simulink model "TPR_Ursino"  (Simulink 7.0)
settings: Solver=ode45  StartTime=0.0  StopTime=10.0  RelTol=1e-3
undefined symbols (not defined in the file or in its folder): Dx, ftas_min, Gas_sleep, initx, toux
settings Model: Creator=CLM  LastModifiedBy=CLM
settings OptimizationCC: BlockReduction=off  BooleanDataType=off
settings DebuggingCC: SaveWithParameterizedLinksMsg=none  SignalResolutionControl=TryResolveAllWithWarning  SolverPrmCheckMsg=none  MultiTaskDSMMsg=warning  MultiTaskCondExecSysMsg=none  StrictBusMsg=None
settings HardwareCC: TargetUnknown=on
settings RTWCC: IncludeERTFirstTime=on
settings GRTTargetCC: TargetFcnLib=ansi_tfl_tmw.mat

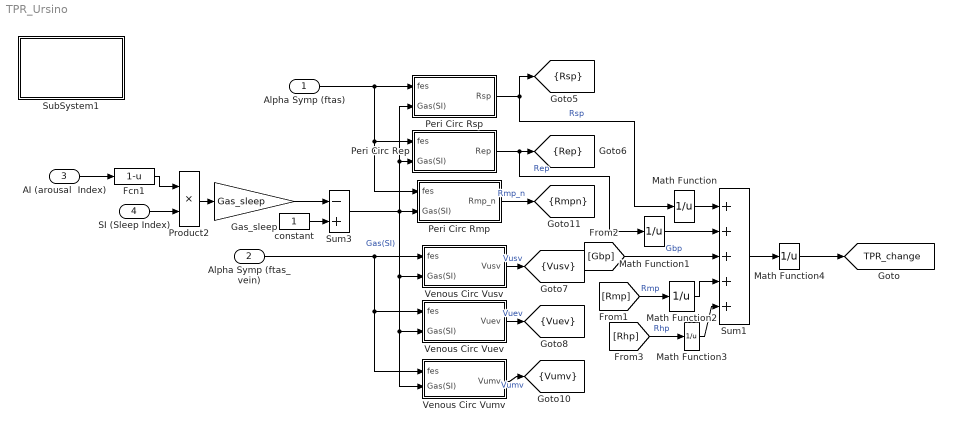
== system TPR_Ursino ==
  Alpha Symp (ftas) : Inport  OutDataType=sfix(16)  OutScaling=2^0
  Alpha Symp (ftas_vein) : Inport  Port=2  OutDataType=sfix(16)  OutScaling=2^0
  AI (arousal  Index) : Inport  Port=3  OutDataType=sfix(16)  OutScaling=2^0
  "SI (Sleep Index) " : Inport  Port=4  OutDataType=sfix(16)  OutScaling=2^0
  Fcn1 : Fcn  Expr=1-u
  Gas_sleep : Gain  Gain=Gas_sleep  ParameterDataType=sfix(16)  ParameterScaling=2^0  OutDataType=sfix(16)  OutScaling=2^0  SaturateOnIntegerOverflow=on
  Math Function{,1..4} (5 alike) : Math  Operator=reciprocal  OutDataType=sfix(16)  OutScaling=2^0  SaturateOnIntegerOverflow=on
  Peri Circ Rep : Subsystem
  Peri Circ Rmp : Subsystem
  Peri Circ Rsp : Subsystem
  Product2 : Product  OutDataType=sfix(16)  OutScaling=2^0  SaturateOnIntegerOverflow=on  InputSameDT=on
  SubSystem1 : Subsystem
      settings: OpenFcn=pneuma_variables
      mask Display: disp('"double click here"\n to load \nTPR_Ursino \ninitial values');
  Sum1 : Sum  Inputs=+++++  OutDataType=sfix(16)  OutScaling=2^0  SaturateOnIntegerOverflow=on  InputSameDT=on
  Sum3 : Sum  Inputs=-+  OutDataType=sfix(16)  OutScaling=2^0  SaturateOnIntegerOverflow=on  InputSameDT=on
  Venous Circ Vuev : Subsystem
  Venous Circ Vumv : Subsystem
  Venous Circ Vusv : Subsystem
  constant : Constant  OutDataType=sfix(16)  OutScaling=2^0
  tag scope: Rep=scoped, Rmpn=scoped, Rsp=scoped, TPR_change=global, Vuev=scoped, Vumv=scoped, Vusv=scoped
  wires:
  AI (arousal  Index)/1 -> Fcn1/1
  "SI (Sleep Index) "/1 -> Product2/2
  Fcn1/1 -> Product2/1
  Product2/1 -> Gas_sleep/1
  constant/1 -> Sum3/2
  Gas_sleep/1 -> Sum3/1
  Peri Circ Rep/1(Rep) -> [Rep], Math Function1/1  "Rep"
  Venous Circ Vusv/1(Vusv) -> [Vusv]  "Vusv"
  Venous Circ Vuev/1(Vuev) -> [Vuev]  "Vuev"
  Peri Circ Rsp/1(Rsp) -> [Rsp], Math Function/1  "Rsp"
  Venous Circ Vumv/1(Vumv) -> [Vumv]  "Vumv"
  Peri Circ Rmp/1(Rmp_n) -> [Rmpn]  "Rmp_n"
  Alpha Symp (ftas)/1 -> Peri Circ Rep/1(fes), Peri Circ Rmp/1(fes), Peri Circ Rsp/1(fes)
  Sum3/1 -> Peri Circ Rsp/2(Gas(SI)), Peri Circ Rep/2(Gas(SI)), Venous Circ Vusv/2(Gas(SI)), Venous Circ Vuev/2(Gas(SI)), Venous Circ Vumv/2(Gas(SI)), Peri Circ Rmp/2(Gas(SI))  "Gas(SI)"
  Alpha Symp (ftas_vein)/1 -> Venous Circ Vusv/1(fes), Venous Circ Vuev/1(fes), Venous Circ Vumv/1(fes)
  Sum1/1 -> Math Function4/1
  [Gbp] -> Sum1/3  "Gbp"
  [Rmp] -> Math Function2/1  "Rmp"
  [Rhp] -> Math Function3/1  "Rhp"
  Math Function/1 -> Sum1/1
  Math Function1/1 -> Sum1/2
  Math Function2/1 -> Sum1/4
  Math Function3/1 -> Sum1/5
  Math Function4/1 -> [TPR_change]

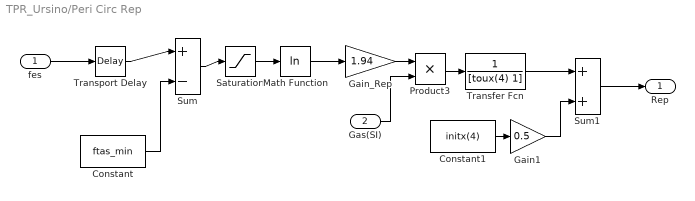
== system TPR_Ursino/Peri Circ Rep ==
  fes : Inport  OutDataType=sfix(16)  OutScaling=2^0
  Gas(SI) : Inport  Port=2  OutDataType=sfix(16)  OutScaling=2^0
  Constant : Constant  Value=ftas_min  OutDataType=sfix(16)  OutScaling=2^0
  Constant1 : Constant  Value=initx(4)  OutDataType=sfix(16)  OutScaling=2^0
  Gain1 : Gain  Gain=0.5  ParameterDataType=sfix(16)  ParameterScaling=2^0  OutDataType=sfix(16)  OutScaling=2^0  SaturateOnIntegerOverflow=on
  Gain_Rep : Gain  Gain=1.94  ParameterDataType=sfix(16)  ParameterScaling=2^0  OutDataType=sfix(16)  OutScaling=2^0  SaturateOnIntegerOverflow=on
  Math Function : Math  Operator=log  OutDataType=sfix(16)  OutScaling=2^0  SaturateOnIntegerOverflow=on
  Product3 : Product  OutDataType=sfix(16)  OutScaling=2^0  SaturateOnIntegerOverflow=on  InputSameDT=on
  Saturation : Saturate  UpperLimit=inf  LowerLimit=1
  Sum : Sum  Inputs=|+-  OutDataType=sfix(16)  OutScaling=2^0  SaturateOnIntegerOverflow=on  InputSameDT=on
  Sum1 : Sum  OutDataType=sfix(16)  OutScaling=2^0  SaturateOnIntegerOverflow=on  InputSameDT=on
  Transfer Fcn : TransferFcn  Denominator=[toux(4) 1]
  Transport Delay : TransportDelay  DelayTime=Dx(4)*0.7  InitialOutput=10  BufferSize=19456
  Rep : Outport  OutDataType=sfix(16)  OutScaling=2^0
  wires:
  Constant1/1 -> Gain1/1
  Sum1/1 -> Rep/1
  Transfer Fcn/1 -> Sum1/1
  Math Function/1 -> Gain_Rep/1
  Saturation/1 -> Math Function/1
  Sum/1 -> Saturation/1
  Constant/1 -> Sum/2
  Transport Delay/1 -> Sum/1
  fes/1 -> Transport Delay/1
  Gas(SI)/1 -> Product3/2
  Gain_Rep/1 -> Product3/1
  Product3/1 -> Transfer Fcn/1
  Gain1/1 -> Sum1/2

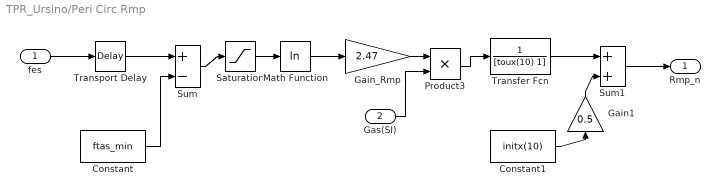
== system TPR_Ursino/Peri Circ Rmp ==
  fes : Inport  OutDataType=sfix(16)  OutScaling=2^0
  Gas(SI) : Inport  Port=2  OutDataType=sfix(16)  OutScaling=2^0
  Constant : Constant  Value=ftas_min  OutDataType=sfix(16)  OutScaling=2^0
  Constant1 : Constant  Value=initx(10)  OutDataType=sfix(16)  OutScaling=2^0
  Gain1 : Gain  Orientation=up  Gain=0.5  ParameterDataType=sfix(16)  ParameterScaling=2^0  OutDataType=sfix(16)  OutScaling=2^0  SaturateOnIntegerOverflow=on
  Gain_Rmp : Gain  Gain=2.47  ParameterDataType=sfix(16)  ParameterScaling=2^0  OutDataType=sfix(16)  OutScaling=2^0  SaturateOnIntegerOverflow=on
  Math Function : Math  Operator=log  OutDataType=sfix(16)  OutScaling=2^0  SaturateOnIntegerOverflow=on
  Product3 : Product  OutDataType=sfix(16)  OutScaling=2^0  SaturateOnIntegerOverflow=on  InputSameDT=on
  Saturation : Saturate  UpperLimit=inf  LowerLimit=1
  Sum : Sum  Inputs=+-  OutDataType=sfix(16)  OutScaling=2^0  SaturateOnIntegerOverflow=on  InputSameDT=on
  Sum1 : Sum  OutDataType=sfix(16)  OutScaling=2^0  SaturateOnIntegerOverflow=on  InputSameDT=on
  Transfer Fcn : TransferFcn  Denominator=[toux(10) 1]
  Transport Delay : TransportDelay  DelayTime=Dx(10)*0.7  InitialOutput=10  BufferSize=19456
  Rmp_n : Outport  OutDataType=sfix(16)  OutScaling=2^0
  wires:
  Constant1/1 -> Gain1/1
  Sum1/1 -> Rmp_n/1
  Transfer Fcn/1 -> Sum1/1
  Math Function/1 -> Gain_Rmp/1
  Saturation/1 -> Math Function/1
  Sum/1 -> Saturation/1
  Constant/1 -> Sum/2
  Transport Delay/1 -> Sum/1
  fes/1 -> Transport Delay/1
  Gas(SI)/1 -> Product3/2
  Gain_Rmp/1 -> Product3/1
  Product3/1 -> Transfer Fcn/1
  Gain1/1 -> Sum1/2

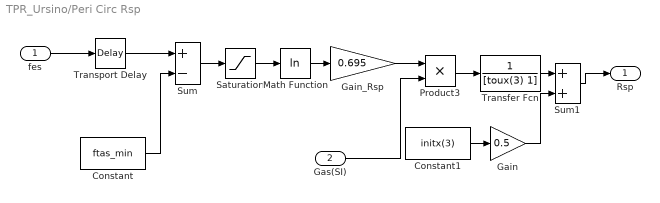
== system TPR_Ursino/Peri Circ Rsp ==
  fes : Inport  OutDataType=sfix(16)  OutScaling=2^0
  Gas(SI) : Inport  Port=2  OutDataType=sfix(16)  OutScaling=2^0
  Constant : Constant  Value=ftas_min  OutDataType=sfix(16)  OutScaling=2^0
  Constant1 : Constant  Value=initx(3)  OutDataType=sfix(16)  OutScaling=2^0
  Gain : Gain  Gain=0.5  ParameterDataType=sfix(16)  ParameterScaling=2^0  OutDataType=sfix(16)  OutScaling=2^0  SaturateOnIntegerOverflow=on
  Gain_Rsp : Gain  Gain=0.695  ParameterDataType=sfix(16)  ParameterScaling=2^0  OutDataType=sfix(16)  OutScaling=2^0  SaturateOnIntegerOverflow=on
  Math Function : Math  Operator=log  OutDataType=sfix(16)  OutScaling=2^0  SaturateOnIntegerOverflow=on
  Product3 : Product  OutDataType=sfix(16)  OutScaling=2^0  SaturateOnIntegerOverflow=on  InputSameDT=on
  Saturation : Saturate  UpperLimit=inf  LowerLimit=1
  Sum : Sum  Inputs=+-  OutDataType=sfix(16)  OutScaling=2^0  SaturateOnIntegerOverflow=on  InputSameDT=on
  Sum1 : Sum  OutDataType=sfix(16)  OutScaling=2^0  SaturateOnIntegerOverflow=on  InputSameDT=on
  Transfer Fcn : TransferFcn  Denominator=[toux(3) 1]
  Transport Delay : TransportDelay  DelayTime=Dx(3)*0.7  InitialOutput=10  BufferSize=19456
  Rsp : Outport  OutDataType=sfix(16)  OutScaling=2^0
  wires:
  fes/1 -> Transport Delay/1
  Transport Delay/1 -> Sum/1
  Constant/1 -> Sum/2
  Sum/1 -> Saturation/1
  Saturation/1 -> Math Function/1
  Math Function/1 -> Gain_Rsp/1
  Transfer Fcn/1 -> Sum1/1
  Sum1/1 -> Rsp/1
  Constant1/1 -> Gain/1
  Gas(SI)/1 -> Product3/2
  Gain_Rsp/1 -> Product3/1
  Product3/1 -> Transfer Fcn/1
  Gain/1 -> Sum1/2

== system TPR_Ursino/SubSystem1 ==

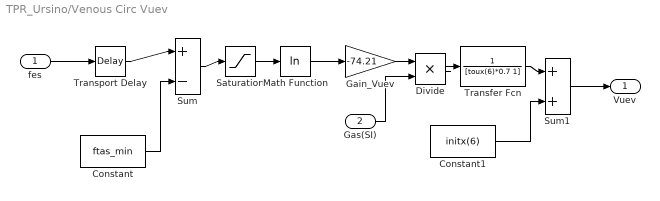
== system TPR_Ursino/Venous Circ Vuev ==
  fes : Inport  OutDataType=sfix(16)  OutScaling=2^0
  Gas(SI) : Inport  Port=2  OutDataType=sfix(16)  OutScaling=2^0
  Constant : Constant  Value=ftas_min  OutDataType=sfix(16)  OutScaling=2^0
  Constant1 : Constant  Value=initx(6)  OutDataType=sfix(16)  OutScaling=2^0
  Divide : Product  Inputs=**  OutDataType=sfix(16)  OutScaling=2^-10
  Gain_Vuev : Gain  Gain=-74.21  ParameterDataType=sfix(16)  ParameterScaling=2^0  OutDataType=sfix(16)  OutScaling=2^0  SaturateOnIntegerOverflow=on
  Math Function : Math  Operator=log  OutDataType=sfix(16)  OutScaling=2^0  SaturateOnIntegerOverflow=on
  Saturation : Saturate  UpperLimit=inf  LowerLimit=1
  Sum : Sum  Inputs=|+-  OutDataType=sfix(16)  OutScaling=2^0  SaturateOnIntegerOverflow=on  InputSameDT=on
  Sum1 : Sum  OutDataType=sfix(16)  OutScaling=2^0  SaturateOnIntegerOverflow=on  InputSameDT=on
  Transfer Fcn : TransferFcn  Denominator=[toux(6)*0.7 1]
  Transport Delay : TransportDelay  DelayTime=Dx(6)*0.7  InitialOutput=10  BufferSize=19456
  Vuev : Outport  OutDataType=sfix(16)  OutScaling=2^0
  wires:
  Constant1/1 -> Sum1/2
  Sum1/1 -> Vuev/1
  Transfer Fcn/1 -> Sum1/1
  Math Function/1 -> Gain_Vuev/1
  Saturation/1 -> Math Function/1
  Sum/1 -> Saturation/1
  Constant/1 -> Sum/2
  Transport Delay/1 -> Sum/1
  fes/1 -> Transport Delay/1
  Gain_Vuev/1 -> Divide/1
  Divide/1 -> Transfer Fcn/1
  Gas(SI)/1 -> Divide/2

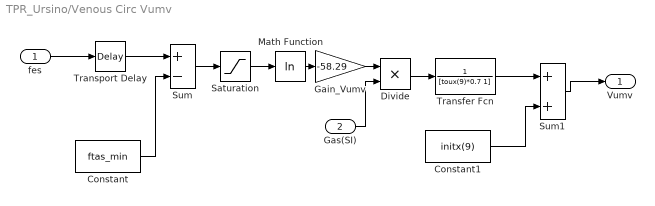
== system TPR_Ursino/Venous Circ Vumv ==
  fes : Inport  OutDataType=sfix(16)  OutScaling=2^0
  Gas(SI) : Inport  Port=2  OutDataType=sfix(16)  OutScaling=2^0
  Constant : Constant  Value=ftas_min  OutDataType=sfix(16)  OutScaling=2^0
  Constant1 : Constant  Value=initx(9)  OutDataType=sfix(16)  OutScaling=2^0
  Divide : Product  Inputs=**  OutDataType=sfix(16)  OutScaling=2^-10
  Gain_Vumv : Gain  Gain=-58.29  ParameterDataType=sfix(16)  ParameterScaling=2^0  OutDataType=sfix(16)  OutScaling=2^0  SaturateOnIntegerOverflow=on
  Math Function : Math  Operator=log  OutDataType=sfix(16)  OutScaling=2^0  SaturateOnIntegerOverflow=on
  Saturation : Saturate  UpperLimit=inf  LowerLimit=1
  Sum : Sum  Inputs=+-  OutDataType=sfix(16)  OutScaling=2^0  SaturateOnIntegerOverflow=on  InputSameDT=on
  Sum1 : Sum  OutDataType=sfix(16)  OutScaling=2^0  SaturateOnIntegerOverflow=on  InputSameDT=on
  Transfer Fcn : TransferFcn  Denominator=[toux(9)*0.7 1]
  Transport Delay : TransportDelay  DelayTime=Dx(9)*0.7  InitialOutput=10  BufferSize=19456
  Vumv : Outport  OutDataType=sfix(16)  OutScaling=2^0
  wires:
  Constant1/1 -> Sum1/2
  Sum1/1 -> Vumv/1
  Transfer Fcn/1 -> Sum1/1
  Math Function/1 -> Gain_Vumv/1
  Saturation/1 -> Math Function/1
  Sum/1 -> Saturation/1
  Constant/1 -> Sum/2
  Transport Delay/1 -> Sum/1
  fes/1 -> Transport Delay/1
  Gas(SI)/1 -> Divide/2
  Gain_Vumv/1 -> Divide/1
  Divide/1 -> Transfer Fcn/1

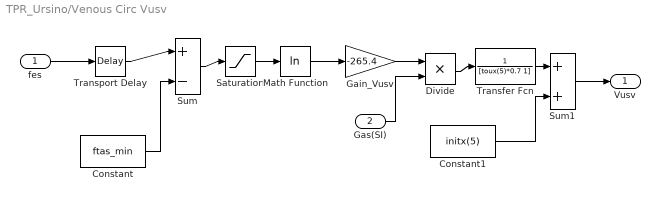
== system TPR_Ursino/Venous Circ Vusv ==
  fes : Inport  OutDataType=sfix(16)  OutScaling=2^0
  Gas(SI) : Inport  Port=2  OutDataType=sfix(16)  OutScaling=2^0
  Constant : Constant  Value=ftas_min  OutDataType=sfix(16)  OutScaling=2^0
  Constant1 : Constant  Value=initx(5)  OutDataType=sfix(16)  OutScaling=2^0
  Divide : Product  Inputs=**  OutDataType=sfix(16)  OutScaling=2^-10
  Gain_Vusv : Gain  Gain=-265.4  ParameterDataType=sfix(16)  ParameterScaling=2^0  OutDataType=sfix(16)  OutScaling=2^0  SaturateOnIntegerOverflow=on
  Math Function : Math  Operator=log  OutDataType=sfix(16)  OutScaling=2^0  SaturateOnIntegerOverflow=on
  Saturation : Saturate  UpperLimit=inf  LowerLimit=1
  Sum : Sum  Inputs=|+-  OutDataType=sfix(16)  OutScaling=2^0  SaturateOnIntegerOverflow=on  InputSameDT=on
  Sum1 : Sum  OutDataType=sfix(16)  OutScaling=2^0  SaturateOnIntegerOverflow=on  InputSameDT=on
  Transfer Fcn : TransferFcn  Denominator=[toux(5)*0.7 1]
  Transport Delay : TransportDelay  DelayTime=Dx(5)*0.7  InitialOutput=10  BufferSize=19456
  Vusv : Outport  OutDataType=sfix(16)  OutScaling=2^0
  wires:
  fes/1 -> Transport Delay/1
  Transport Delay/1 -> Sum/1
  Constant/1 -> Sum/2
  Sum/1 -> Saturation/1
  Saturation/1 -> Math Function/1
  Math Function/1 -> Gain_Vusv/1
  Transfer Fcn/1 -> Sum1/1
  Sum1/1 -> Vusv/1
  Constant1/1 -> Sum1/2
  Gas(SI)/1 -> Divide/2
  Gain_Vusv/1 -> Divide/1
  Divide/1 -> Transfer Fcn/1
